simulink model "diagram"  (R2024b)
settings: Solver=FixedStepAuto  StartTime=0.0  StopTime=10.0  FixedStep=0.01  RelTol=1e-3
settings Model: Creator=jz74  LastModifiedBy=jz74

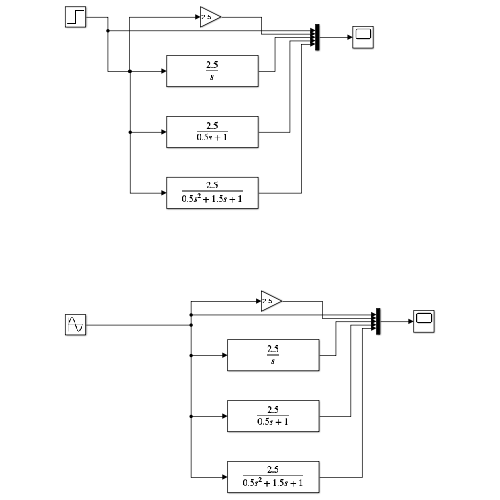
[thumbnail: Simulink's stored preview of the top-level diagram]
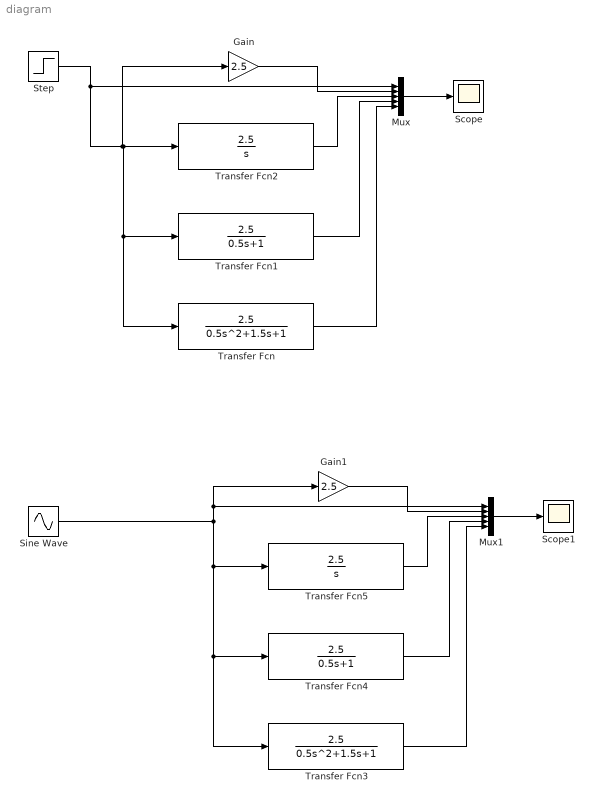
== system diagram ==
  Gain : Gain  Gain=2.5
  Gain1 : Gain  Gain=2.5
  Mux : Mux  Inputs=5
  Mux1 : Mux  Inputs=5
  Scope : Scope
  Scope1 : Scope
  Sine Wave : Sin  Frequency=5  SampleTime=0
  Step : Step  SampleTime=0
  Transfer Fcn : TransferFcn  Numerator=[2.5]  Denominator=[0.5 1.5 1]
  Transfer Fcn1 : TransferFcn  Numerator=[2.5]  Denominator=[0.5 1]
  Transfer Fcn2 : TransferFcn  Numerator=[2.5]  Denominator=[1 0]
  Transfer Fcn3 : TransferFcn  Numerator=[2.5]  Denominator=[0.5 1.5 1]
  Transfer Fcn4 : TransferFcn  Numerator=[2.5]  Denominator=[0.5 1]
  Transfer Fcn5 : TransferFcn  Numerator=[2.5]  Denominator=[1 0]
  wires:
  Gain/1 -> Mux/2
  Transfer Fcn2/1 -> Mux/3
  Transfer Fcn1/1 -> Mux/4
  Transfer Fcn/1 -> Mux/5
  Mux/1 -> Scope/1
  Step/1 -> Gain/1, Transfer Fcn/1, Transfer Fcn1/1, Transfer Fcn2/1, Mux/1
  Transfer Fcn3/1 -> Mux1/5
  Mux1/1 -> Scope1/1
  Transfer Fcn4/1 -> Mux1/4
  Sine Wave/1 -> Gain1/1, Mux1/1, Transfer Fcn3/1, Transfer Fcn4/1, Transfer Fcn5/1
  Gain1/1 -> Mux1/2
  Transfer Fcn5/1 -> Mux1/3
